simulink model "PuttingItAllTogether"  (R2020b)
settings: Solver=VariableStepAuto  StartTime=0.0  StopTime=10.0  RelTol=1e-5
values from neighbouring files (symbols this model uses):
  den = [SIM.R*SIM.C, 1]    [TestingFunctionHandles.m]
  num = [SIM.R]    [TestingFunctionHandles.m]
settings Model: Creator=tyevans  LastModifiedBy=tyevans

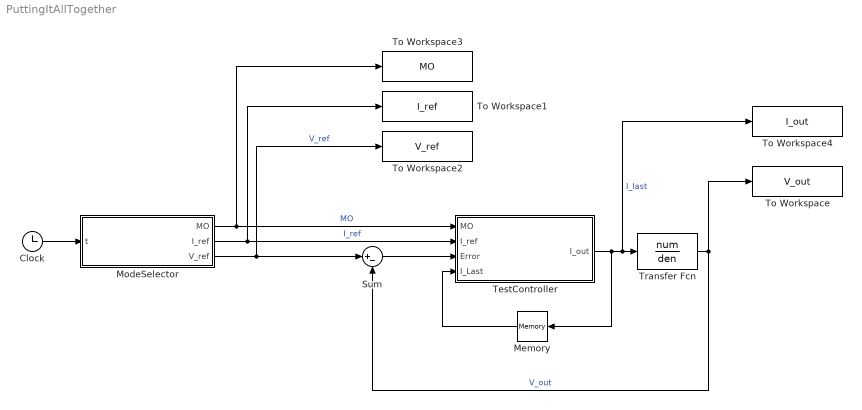
== system PuttingItAllTogether ==
  Clock : Clock
  Memory : Memory  InheritSampleTime=on
  ModeSelector : MATLAB Function  TreatAsAtomicUnit=on
  Sum : Sum  Inputs=|+-
  TestController : MATLAB Function  TreatAsAtomicUnit=on
  To Workspace : ToWorkspace  VariableName=V_out  SampleTime=-1
  To Workspace1 : ToWorkspace  VariableName=I_ref  SampleTime=-1
  To Workspace2 : ToWorkspace  VariableName=V_ref  SampleTime=-1
  To Workspace3 : ToWorkspace  VariableName=MO  SampleTime=-1
  To Workspace4 : ToWorkspace  VariableName=I_out  SampleTime=-1
  Transfer Fcn : TransferFcn  Numerator=num  Denominator=den
  wires:
  Clock/1 -> ModeSelector/1(t)
  ModeSelector/1(MO) -> To Workspace3/1, TestController/1(MO)  "MO"
  ModeSelector/2(I_ref) -> To Workspace1/1, TestController/2(I_ref)  "I_ref"
  ModeSelector/3(V_ref) -> Sum/1, To Workspace2/1  "V_ref"
  Transfer Fcn/1 -> Sum/2, To Workspace/1  "V_out"
  TestController/1(I_out) -> Memory/1, To Workspace4/1, Transfer Fcn/1  "I_last"
  Sum/1 -> TestController/3(Error)
  Memory/1 -> TestController/4(I_Last)

== matlab function PuttingItAllTogether/TestController ==
  data: MO input; I_out output; I_ref input; Error input; I_Last input
function I_out = TestController(MO, I_ref, Error, I_Last)
if MO == 1 % CC Mode
    I_out = I_ref;
elseif MO == 2 % CV Mode
    K_p = 0.25;
    I_out = K_p * Error + I_Last;
else
    I_out = 0;
end
end

== matlab function PuttingItAllTogether/ModeSelector ==
  data: t input; MO output; I_ref output; V_ref output; SIM parameter
function [MO,I_ref,V_ref] = ModeSelector(t, SIM)
% Initialize Outputs Data Types
MO    = 1;
I_ref = 0.0;
V_ref = 0.0;

% Call Matlab Function
coder.extrinsic('myMode');
[MO,I_ref,V_ref] = myMode(t,SIM);
end
